simulink model "VF"  (R2016b)
settings: Solver=VariableStepAuto  StartTime=0.0  StopTime=10.0  RelTol=1e-3
undefined symbols (not defined in the file): DiscIntNeverNeededParam
libraries: hdlsllib x3
settings Model: Creator=paul.rogers  LastModifiedBy=paul.rogers
settings OptimizationCC: BlockReduction=off  ConditionallyExecuteInputs=off  DefaultParameterBehavior=Inlined
settings DebuggingCC: AlgebraicLoopMsg=error  SingleTaskRateTransMsg=error
settings HardwareCC: ProdBitPerPointer=32  ProdBitPerSizeT=32  ProdBitPerPtrDiffT=32  ProdLargestAtomicFloat=None  ProdIntDivRoundTo=Undefined  ProdEndianess=Unspecified  ProdWordSize=32  ProdHWDeviceType=ASIC/FPGA->ASIC/FPGA  ProdEqTarget=off

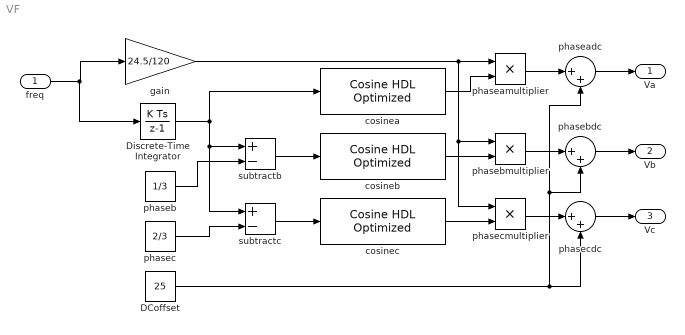
== system VF ==
  freq : Inport  OutDataTypeStr=fixdt(1,16,12)  Unit=Hz
  DCoffset : Constant  Value=25  OutDataTypeStr=uint16  SampleTime=-1
  Discrete-Time Integrator : DiscreteIntegrator  SampleTime=0.000000081  OutDataTypeStr=fixdt(1,64,35)  ICPrevOutput=DiscIntNeverNeededParam  ICPrevScaledInput=DiscIntNeverNeededParam
  cosinea : hdlsllib/Lookup Tables/Cosine HDL Optimized  OutputFormula=cos(2*pi*u)  NumDataPoints=2^12  TableDataTypeStr=fixdt(1,50,42)  SimulateLUTROMDelay=off
  cosineb : hdlsllib/Lookup Tables/Cosine HDL Optimized  OutputFormula=cos(2*pi*u)  NumDataPoints=2^12  TableDataTypeStr=fixdt(1,50,42)  SimulateLUTROMDelay=off
  cosinec : hdlsllib/Lookup Tables/Cosine HDL Optimized  OutputFormula=cos(2*pi*u)  NumDataPoints=2^12  TableDataTypeStr=fixdt(1,50,42)  SimulateLUTROMDelay=off
  gain : Gain  Gain=24.5/120  ParamDataTypeStr=fixdt(1,16,12)
  phaseadc : Sum  Inputs=|++
  phaseamultiplier : Product
  phaseb : Constant  Value=1/3  OutDataTypeStr=fixdt(1,16,12)  SampleTime=0.000000081
  phasebdc : Sum  Inputs=|++
  phasebmultiplier : Product
  phasec : Constant  Value=2/3  OutDataTypeStr=fixdt(1,16,12)  SampleTime=0.000000081
  phasecdc : Sum  Inputs=|++
  phasecmultiplier : Product
  subtractb : Sum  Inputs=+-
  subtractc : Sum  Inputs=+-
  Va : Outport
  Vb : Outport  Port=2
  Vc : Outport  Port=3
  wires:
  phasec/1 -> subtractc/2
  cosinea/1 -> phaseamultiplier/2
  phaseamultiplier/1 -> phaseadc/1
  Discrete-Time Integrator/1 -> subtractc/1, subtractb/1, cosinea/1
  phasebmultiplier/1 -> phasebdc/1
  gain/1 -> phaseamultiplier/1, phasecmultiplier/1, phasebmultiplier/1
  cosineb/1 -> phasebmultiplier/2
  cosinec/1 -> phasecmultiplier/2
  phasecmultiplier/1 -> phasecdc/1
  subtractc/1 -> cosinec/1
  phaseb/1 -> subtractb/2
  subtractb/1 -> cosineb/1
  freq/1 -> Discrete-Time Integrator/1, gain/1
  DCoffset/1 -> phasecdc/2, phaseadc/2, phasebdc/2
  phasecdc/1 -> Vc/1
  phasebdc/1 -> Vb/1
  phaseadc/1 -> Va/1
